simulink model "lorenz_sim"  (Simulink 6.3)
settings: Solver=ode4  StartTime=0.0  StopTime=5  FixedStep=0.01  RelTol=1e-3
values from neighbouring files (symbols this model uses):
  b = 8/3    (= 2.66666666667)    [fix_r_lya.m]    (also in test_wolf.m)
  delt = (max_d-min_d)/ss    [G_P.m]    (also in fix_r_lya.m = 10; test_wolf.m = 10)
  r = size(X,1)    [DMD1.m]    (also in G_P.m = min_d+k*delt; fix_r_lya.m = 114; test_wolf.m = r_test(i))
  x0 = 1    [fix_r_lya.m]    (also in test_wolf.m; traj.mat = [0.0916520213601 0.0923186171986 0.0929633815691 0.093585608)
  y0 = 1    [fix_r_lya.m]    (also in test_wolf.m)
  z0 = (targetdata(:,1)-xautofull(:,1))/ep    [LQRwdz3.m]    (also in LQRwdz3_QR.m; LQRwdz4.m; fix_r_lya.m = 1; test_wolf.m = 1)
settings Model: ModifiedByFormat=zhl_chosenone  LastModifiedBy=zhl_chosenone

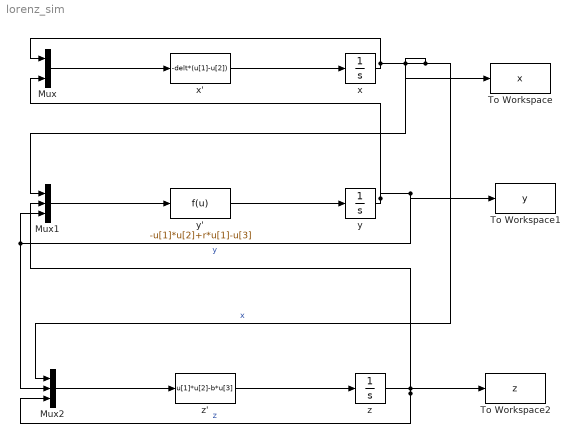
== system lorenz_sim ==
  Mux : Mux  Inputs=2
  Mux1 : Mux  Inputs=3
  Mux2 : Mux  Inputs=3
  To Workspace : ToWorkspace  VariableName=x  SampleTime=-1  SaveFormat=Array
  To Workspace1 : ToWorkspace  VariableName=y  SampleTime=-1  SaveFormat=Array
  To Workspace2 : ToWorkspace  VariableName=z  SampleTime=-1  SaveFormat=Array
  x : Integrator  InitialCondition=x0
  x' : Fcn  Expr=-delt*(u[1]-u[2])
  y : Integrator  InitialCondition=y0
  y' : Fcn  Expr=-u[1]*u[2]+r*u[1]-u[3]
  z : Integrator  InitialCondition=z0
  z' : Fcn  Expr=u[1]*u[2]-b*u[3]
  wires:
  Mux/1 -> x'/1
  x'/1 -> x/1
  Mux1/1 -> y'/1
  y'/1 -> y/1
  Mux2/1 -> z'/1
  z'/1 -> z/1
  x/1 -> Mux/1, Mux1/1, Mux2/1, To Workspace/1  "x"
  y/1 -> Mux/2, Mux1/3, Mux2/2, To Workspace1/1  "y"
  z/1 -> Mux1/2, Mux2/3, To Workspace2/1  "z"
